simulink model "tp352185"  (Simulink 3.0)
settings: Solver=ode1  SolverMode=SingleTasking  StartTime=0.0  StopTime=t_sim  FixedStep=Ts  RelTol=1e-3
values from neighbouring files (symbols this model uses):
  arw_on = 1    [prech_light.mat]
  I = 0.5    [prech_light.mat]
  P = (1-lambda)/(Ks*Ts)    [init_PI1_disc_windupless.m]    (also in prech_light.mat = 2)
  t_prep = 0    [init_io_char_up_oloop.m]    (also in prech_light.mat = 40)
  Ts = 0.2    [init_I0_cont.m]    (also in init_PI1_disc_windupless.m = Td*2; init_io_char_up_oloop.m = 0.1; prech_light.mat)
  u_step = 4    [prech_light.mat]
  Umax = 5    [init_I0_cont.m]    (also in init_PI1_disc_windupless.m; init_io_char_up_oloop.m; prech_light.mat)
  Umin = 0    [init_I0_cont.m]    (also in init_PI1_disc_windupless.m; init_io_char_up_oloop.m; prech_light.mat)
  w = [0 .1 .2 .3 .4 .5 .6 .7 .8 .9 1 ]*u_range + Umin    [init_io_char_up_oloop.m]    (also in prech_light.mat = 20)
libraries: udaq28LT_lib x1
settings Model: LastModifiedBy=mato  SaveFormat=Matrix  BooleanDataType=on

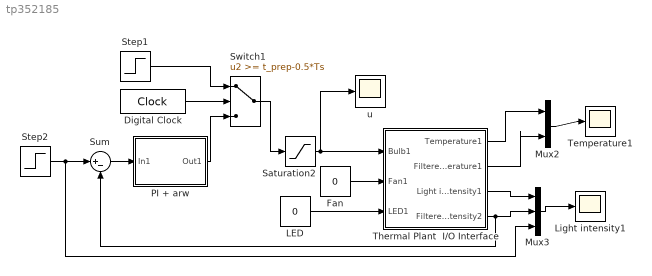
== system tp352185 ==
  Digital Clock : DigitalClock  SampleTime=Ts
  Fan : Constant  Value=0
  LED : Constant  Value=0
  Light intensity1 : Scope
      settings: TickLabels=on  TimeRange=30  YMin=0  YMax=100  SaveName=yl  DataFormat=Matrix
  Mux2 : Mux  Inputs=2
  Mux3 : Mux  Inputs=3
  PI + arw : Subsystem
  Saturation2 : Saturate  UpperLimit=Umax  LowerLimit=Umin
  Step1 : Step  Time=0  Before=0  After=u_step  SampleTime=Ts
  Step2 : Step  Time=0  Before=0  After=w  SampleTime=Ts
  Sum : Sum  Inputs=|+-  SaturateOnIntegerOverflow=on
  Switch1 : Switch  Threshold=t_prep-0.5*Ts
  Temperature1 : Scope
      settings: TickLabels=on  TimeRange=30  YMin=15  YMax=50  SaveName=yt  DataFormat=Matrix
  Thermal Plant  I/O Interface : Subsystem
      mask Display: disp('Thermo-optical\nPlant\nI/O Interface')
  u : Scope
      settings: TimeRange=220  YMin=0  YMax=5.5  SaveName=u  DataFormat=Matrix  Decimation=10  SampleInput=on  SampleTime=Ts
  wires:
  Saturation2/1 -> u/1, Thermal Plant  I/O Interface/1(Bulb1)
  Digital Clock/1 -> Switch1/2
  Switch1/1 -> Saturation2/1
  Step1/1 -> Switch1/1
  PI + arw/1(Out1) -> Switch1/3
  Sum/1 -> PI + arw/1(In1)
  Step2/1 -> Sum/1, Mux3/3
  Mux2/1 -> Temperature1/1
  Mux3/1 -> Light intensity1/1
  Fan/1 -> Thermal Plant  I/O Interface/2(Fan1)
  LED/1 -> Thermal Plant  I/O Interface/3(LED1)
  Thermal Plant  I/O Interface/1(Temperature1) -> Mux2/1
  Thermal Plant  I/O Interface/2(Filtered  temperature1) -> Mux2/2
  Thermal Plant  I/O Interface/3(Light intensity1) -> Mux3/1
  Thermal Plant  I/O Interface/4(Filtered  light intensity2) -> Mux3/2, Sum/2

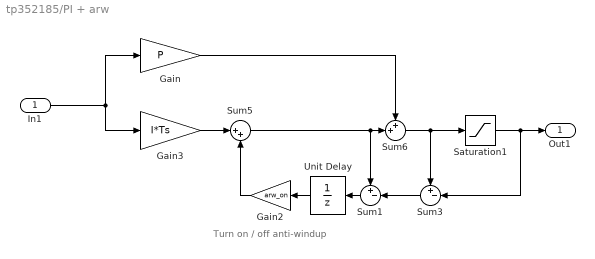
== system tp352185/PI + arw ==
  note: Turn on / off
      | anti-windup
  In1 : Inport  Port=1  PortWidth=-1  SampleTime=-1  DataType=auto
      settings: SignalType=auto
  Gain : Gain  Gain=P  SaturateOnIntegerOverflow=on
  Gain2 : Gain  Orientation=left  Gain=arw_on  SaturateOnIntegerOverflow=on
  Gain3 : Gain  Gain=I*Ts  SaturateOnIntegerOverflow=on
  Saturation1 : Saturate  UpperLimit=Umax  LowerLimit=Umin
  Sum1 : Sum  Orientation=left  Inputs=+-|  SaturateOnIntegerOverflow=on
  Sum3 : Sum  Orientation=left  Inputs=+-|  SaturateOnIntegerOverflow=on
  Sum5 : Sum  Inputs=|++  SaturateOnIntegerOverflow=on
  Sum6 : Sum  Inputs=++|  SaturateOnIntegerOverflow=on
  Unit Delay : UnitDelay  Orientation=left  X0=0  SampleTime=Ts
  Out1 : Outport  Port=1
  wires:
  Sum3/1 -> Sum1/2
  Sum1/1 -> Unit Delay/1
  Gain3/1 -> Sum5/1
  Unit Delay/1 -> Gain2/1
  Sum6/1 -> Sum3/1, Saturation1/1
  Saturation1/1 -> Sum3/2, Out1/1
  In1/1 -> Gain/1, Gain3/1
  Sum5/1 -> Sum1/1, Sum6/2
  Gain/1 -> Sum6/1
  Gain2/1 -> Sum5/2

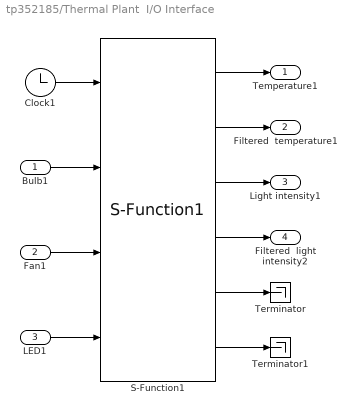
== system tp352185/Thermal Plant  I/O Interface ==
  Bulb1 : Inport  Port=1  PortWidth=-1  SampleTime=-1  DataType=auto
      settings: SignalType=auto
  Fan1 : Inport  Port=2  PortWidth=-1  SampleTime=-1  DataType=auto
      settings: SignalType=auto
  LED1 : Inport  Port=3  PortWidth=-1  SampleTime=-1  DataType=auto
      settings: SignalType=auto
  Clock1 : Clock
      settings: DisplayTime=off  Decimation=10
  S-Function1 : udaq28LT_lib/S-Function1  Priority=1  com_port=COM3  Ts=Ts  events_ot=2  rd_timeout=Ts/2*1000  matlab_prior=ABOVE_NORMAL_PRIORITY  warning=on  printout=off
  Terminator : Terminator
  Terminator1 : Terminator
  Temperature1 : Outport  Port=1
  Filtered  temperature1 : Outport  Port=2
  Light intensity1 : Outport  Port=3
  Filtered  light intensity2 : Outport  Port=4
  wires:
  S-Function1/1 -> Temperature1/1
  S-Function1/2 -> Filtered  temperature1/1
  Clock1/1 -> S-Function1/1
  Bulb1/1 -> S-Function1/2
  Fan1/1 -> S-Function1/3
  S-Function1/3 -> Light intensity1/1
  S-Function1/4 -> Filtered  light intensity2/1
  S-Function1/5 -> Terminator/1
  S-Function1/6 -> Terminator1/1
  LED1/1 -> S-Function1/4
